simulink library "lib_Gimbal_Ctrl"  (R2019a)
settings: Solver=VariableStepAuto  StartTime=0.0  StopTime=10.0  RelTol=1e-3
undefined symbols (not defined in the file or in its folder): FT_HWI_CC_Data, HIL_Data, Standard_Devices, UDP_Protocol
libraries: simulink x19, sldrtlib x2
(part 2 of 2)

== system lib_Gimbal_Ctrl/Gimbel_Ctrl/Gimbal_Controller/Controller/Voltage_Limitations/If Action limit_pitch ==
  In1 : Inport
  Action Port : ActionPort
  Limit_Voltage_Pitch : Saturate  UpperLimit=Gimbal_Ctrl.PitchCmdMaxVolt  LowerLimit=-Gimbal_Ctrl.PitchCmdMaxVolt
  Out1 : Outport
  wires:
  In1/1 -> Limit_Voltage_Pitch/1
  Limit_Voltage_Pitch/1 -> Out1/1

== system lib_Gimbal_Ctrl/Gimbel_Ctrl/Gimbal_Controller/Controller/Voltage_Limitations/If Action limit_roll ==
  In1 : Inport
  Action Port : ActionPort
  Limit_Voltage_Roll : Saturate  UpperLimit=Gimbal_Ctrl.RollCmdMaxVolt  LowerLimit=-Gimbal_Ctrl.RollCmdMaxVolt
  Out1 : Outport
  wires:
  In1/1 -> Limit_Voltage_Roll/1
  Limit_Voltage_Roll/1 -> Out1/1

== system lib_Gimbal_Ctrl/Gimbel_Ctrl/Gimbal_Controller/Controller/Voltage_Limitations/If Action limit_yaw ==
  In1 : Inport
  Action Port : ActionPort
  Limit_Voltage_Yaw : Saturate  UpperLimit=Gimbal_Ctrl.YawCmdMaxVolt  LowerLimit=-Gimbal_Ctrl.YawCmdMaxVolt
  Out1 : Outport
  wires:
  In1/1 -> Limit_Voltage_Yaw/1
  Limit_Voltage_Yaw/1 -> Out1/1

== system lib_Gimbal_Ctrl/Gimbel_Ctrl/Gimbal_Controller/Controller/Voltage_Limitations/If Action pass_pitch ==
  In1 : Inport
  Action Port : ActionPort
  Out1 : Outport
  wires:
  In1/1 -> Out1/1

== system lib_Gimbal_Ctrl/Gimbel_Ctrl/Gimbal_Controller/Controller/Voltage_Limitations/If Action pass_roll ==
  In1 : Inport
  Action Port : ActionPort
  Out1 : Outport
  wires:
  In1/1 -> Out1/1

== system lib_Gimbal_Ctrl/Gimbel_Ctrl/Gimbal_Controller/Controller/Voltage_Limitations/If Action pass_yaw ==
  In1 : Inport
  Action Port : ActionPort
  Out1 : Outport
  wires:
  In1/1 -> Out1/1

== system lib_Gimbal_Ctrl/Gimbel_Ctrl/Gimbal_Controller/Controller/Controller_Pitch/Limits/Enabled adapt ==
  vel : Inport
  upper_limit : Inport  Port=2
  lower_limit : Inport  Port=3
  Enable : EnablePort
  Abs : Abs
  Add : Sum  Inputs=+-
  Constant : Constant  Value=Gimbal_Ctrl.Pitch_hard_limit_vel
  Constant1 : Constant  Value=Gimbal_Ctrl.Pitch_limit_adaption_coef-1
  Divide : Product  Inputs=*/
  Gain : Gain  Gain=Gimbal_Ctrl.Pitch_limit_adaption_coef
  Product : Product
  Product1 : Product
  upper_limit_adapted : Outport
  lower_limit_adapted : Outport  Port=2
  wires:
  Constant/1 -> Abs/1
  Abs/1 -> Divide/1
  vel/1 -> Divide/2
  Divide/1 -> Gain/1
  Gain/1 -> Add/1
  Constant1/1 -> Add/2
  upper_limit/1 -> Product/2
  Add/1 -> Product/1, Product1/1
  Product/1 -> upper_limit_adapted/1
  lower_limit/1 -> Product1/2
  Product1/1 -> lower_limit_adapted/1

== system lib_Gimbal_Ctrl/Gimbel_Ctrl/Gimbal_Controller/Controller/Controller_Pitch/Limits/Enabled pass ==
  upper_limit : Inport
  lower_limit : Inport  Port=2
  Enable : EnablePort
  upper_limit_pass : Outport
  lower_limit_pass : Outport  Port=2
  wires:
  upper_limit/1 -> upper_limit_pass/1
  lower_limit/1 -> lower_limit_pass/1

== system lib_Gimbal_Ctrl/Gimbel_Ctrl/Gimbal_Controller/Controller/Controller_Pitch/PID_Controller_Dynamic_Limits/Saturation ==
  upper_limit : Inport
  lower_limit : Inport  Port=2
  in : Inport  Port=3
  Enable : EnablePort
  Saturation Dynamic : simulink/Discontinuities/Saturation Dynamic  OutMin=[]  OutMax=[]  OutDataTypeStr=Inherit: Same as second input  OutDataType=fixdt(1, 16)  OutScaling=2^-10  DoSatur=off
  out : Outport
  wires:
  in/1 -> Saturation Dynamic/2
  Saturation Dynamic/1 -> out/1
  lower_limit/1 -> Saturation Dynamic/3
  upper_limit/1 -> Saturation Dynamic/1

== system lib_Gimbal_Ctrl/Gimbel_Ctrl/Gimbal_Controller/Controller/Controller_Pitch/PID_Controller_Dynamic_Limits/pass ==
  in : Inport
  Enable : EnablePort
  out : Outport
  wires:
  in/1 -> out/1

== system lib_Gimbal_Ctrl/Gimbel_Ctrl/Gimbal_Controller/Controller/Controller_Roll/Limits/Enabled adapt ==
  vel : Inport
  upper_limit : Inport  Port=2
  lower_limit : Inport  Port=3
  Enable : EnablePort
  Abs : Abs
  Add : Sum  Inputs=+-
  Constant : Constant  Value=Gimbal_Ctrl.Roll_hard_limit_vel
  Constant1 : Constant  Value=Gimbal_Ctrl.Roll_limit_adaption_coef-1
  Divide : Product  Inputs=*/
  Gain : Gain  Gain=Gimbal_Ctrl.Roll_limit_adaption_coef
  Product : Product
  Product1 : Product
  upper_limit_adapted : Outport
  lower_limit_adapted : Outport  Port=2
  wires:
  Constant/1 -> Abs/1
  Abs/1 -> Divide/1
  vel/1 -> Divide/2
  Divide/1 -> Gain/1
  Gain/1 -> Add/1
  Constant1/1 -> Add/2
  upper_limit/1 -> Product/2
  Add/1 -> Product/1, Product1/1
  Product/1 -> upper_limit_adapted/1
  lower_limit/1 -> Product1/2
  Product1/1 -> lower_limit_adapted/1

== system lib_Gimbal_Ctrl/Gimbel_Ctrl/Gimbal_Controller/Controller/Controller_Roll/Limits/Enabled pass ==
  upper_limit : Inport
  lower_limit : Inport  Port=2
  Enable : EnablePort
  upper_limit_pass : Outport
  lower_limit_pass : Outport  Port=2
  wires:
  upper_limit/1 -> upper_limit_pass/1
  lower_limit/1 -> lower_limit_pass/1

== system lib_Gimbal_Ctrl/Gimbel_Ctrl/Gimbal_Controller/Controller/Controller_Roll/PID_Controller_Dynamic_Limits/Saturation ==
  upper_limit : Inport
  lower_limit : Inport  Port=2
  in : Inport  Port=3
  Enable : EnablePort
  Saturation Dynamic : simulink/Discontinuities/Saturation Dynamic  OutMin=[]  OutMax=[]  OutDataTypeStr=Inherit: Same as second input  OutDataType=fixdt(1, 16)  OutScaling=2^-10  DoSatur=off
  out : Outport
  wires:
  in/1 -> Saturation Dynamic/2
  Saturation Dynamic/1 -> out/1
  lower_limit/1 -> Saturation Dynamic/3
  upper_limit/1 -> Saturation Dynamic/1

== system lib_Gimbal_Ctrl/Gimbel_Ctrl/Gimbal_Controller/Controller/Controller_Roll/PID_Controller_Dynamic_Limits/pass ==
  in : Inport
  Enable : EnablePort
  out : Outport
  wires:
  in/1 -> out/1

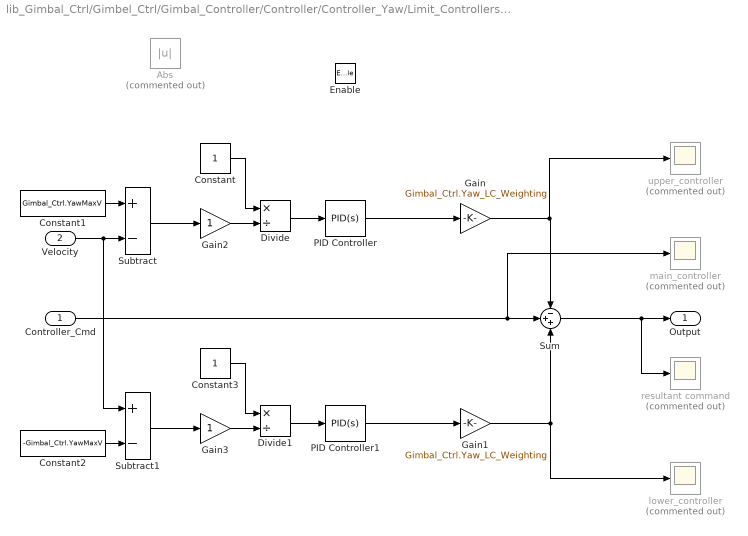
== system lib_Gimbal_Ctrl/Gimbel_Ctrl/Gimbal_Controller/Controller/Controller_Yaw/Limit_Controllers/Control_Limits ==
  Controller_Cmd : Inport
  Velocity : Inport  Port=2
  Enable : EnablePort
  Abs : Abs  Commented=on
  Constant : Constant
  Constant1 : Constant  Value=Gimbal_Ctrl.YawMaxV
  Constant2 : Constant  Value=-Gimbal_Ctrl.YawMaxV
  Constant3 : Constant
  Divide : Product  Inputs=*/
  Divide1 : Product  Inputs=*/
  Gain : Gain  Gain=Gimbal_Ctrl.Yaw_LC_Weighting
  Gain1 : Gain  Gain=Gimbal_Ctrl.Yaw_LC_Weighting
  Gain2 : Gain
  Gain3 : Gain
  PID Controller : simulink/Continuous/PID Controller  Controller=PID  Form=Parallel  TimeDomain=Continuous-time  SampleTime=-1  IntegratorMethod=Forward Euler  FilterMethod=Forward Euler  ControllerParametersSource=internal  P=Gimbal_Ctrl.Yaw_LC_Proportional_Gain  I=Gimbal_Ctrl.Yaw_LC_Integral_Gain  D=Gimbal_Ctrl.Yaw_LC_Derivative_Gain  UseFilter=on  N=100  TunerSelectOption=Transfer Function Based (PID Tuner App)  InitialConditionSource=internal  InitialConditionForIntegrator=0  InitialConditionForFilter=0  DifferentiatorICPrevScaledInput=0  ExternalReset=none  TrackingMode=off  Kt=1  LimitOutput=on  UpperSaturationLimit=20  LowerSaturationLimit=-20  LinearizeAsGain=on  AntiWindupMode=back-calculation  Kb=1  POutMin=[]  POutMax=[]  IOutMin=[]  IOutMax=[]  DOutMin=[]  DOutMax=[]  NOutMin=[]  NOutMax=[]  SumOutMin=[]  SumOutMax=[]  SaturationOutMin=[]  SaturationOutMax=[]  PParamMin=[]  PParamMax=[]  IParamMin=[]  IParamMax=[]  DParamMin=[]  DParamMax=[]  NParamMin=[]  NParamMax=[]  KbParamMin=[]  KbParamMax=[]  KtParamMin=[]  KtParamMax=[]  KbOutMin=[]  KbOutMax=[]  KtOutMin=[]  KtOutMax=[]  IntegratorOutMin=[]  IntegratorOutMax=[]  FilterOutMin=[]  FilterOutMax=[]  SumI1OutMin=[]  SumI1OutMax=[]  SumI2OutMin=[]  SumI2OutMax=[]  SumI3OutMin=[]  SumI3OutMax=[]  SumI4OutMin=[]  SumI4OutMax=[]  SumDOutMin=[]  SumDOutMax=[]  DifferentiatorOutMin=[]  DifferentiatorOutMax=[]  FilterDiffOutCoefMin=[]  FilterDiffOutCoefMax=[]  ReciprocalOutMin=[]  ReciprocalOutMax=[]  SumDenOutMin=[]  SumDenOutMax=[]  SumNumOutMin=[]  SumNumOutMax=[]  DivideOutMin=[]  DivideOutMax=[]  IntegratorContinuousStateAttributes=''  IntegratorStateMustResolveToSignalObject=off  IntegratorRTWStateStorageClass=Auto  FilterContinuousStateAttributes=''  FilterStateMustResolveToSignalObject=off  FilterRTWStateStorageClass=Auto  ParallelPVariant=InternalParameters  IdealPVariant=Disabled  IVariant=InternalParameters  DVariant=InternalParameters  IntegratorVariant=Continuous  SatVariant=Enabled  AWVariant=BackCalculation  PCopyVariant=Disabled  TRVariant=Disabled  FdbkBlocksVariant=Forward  IdealPFdbkVariant=Disabled  SatFdbkVariant=Disabled  DerivativeFilterVariant=ContFilter  NVariant=InternalParameters  NCopyVariant=Disabled  FilterICVariant=InternalICsFilter  IntegratorICVariant=InternalICs  ExternalResetVariant=Disabled  TRSumVariant=Passthrough  SumFdbkVariant=Disabled  SumVariant=Sum_PID
  PID Controller1 : simulink/Continuous/PID Controller  Controller=PID  Form=Parallel  TimeDomain=Continuous-time  SampleTime=-1  IntegratorMethod=Forward Euler  FilterMethod=Forward Euler  ControllerParametersSource=internal  P=Gimbal_Ctrl.Yaw_LC_Proportional_Gain  I=Gimbal_Ctrl.Yaw_LC_Integral_Gain  D=Gimbal_Ctrl.Yaw_LC_Derivative_Gain  UseFilter=on  N=100  TunerSelectOption=Transfer Function Based (PID Tuner App)  InitialConditionSource=internal  InitialConditionForIntegrator=0  InitialConditionForFilter=0  DifferentiatorICPrevScaledInput=0  ExternalReset=none  TrackingMode=off  Kt=1  LimitOutput=on  UpperSaturationLimit=20  LowerSaturationLimit=-20  LinearizeAsGain=off  AntiWindupMode=back-calculation  Kb=1  POutMin=[]  POutMax=[]  IOutMin=[]  IOutMax=[]  DOutMin=[]  DOutMax=[]  NOutMin=[]  NOutMax=[]  SumOutMin=[]  SumOutMax=[]  SaturationOutMin=[]  SaturationOutMax=[]  PParamMin=[]  PParamMax=[]  IParamMin=[]  IParamMax=[]  DParamMin=[]  DParamMax=[]  NParamMin=[]  NParamMax=[]  KbParamMin=[]  KbParamMax=[]  KtParamMin=[]  KtParamMax=[]  KbOutMin=[]  KbOutMax=[]  KtOutMin=[]  KtOutMax=[]  IntegratorOutMin=[]  IntegratorOutMax=[]  FilterOutMin=[]  FilterOutMax=[]  SumI1OutMin=[]  SumI1OutMax=[]  SumI2OutMin=[]  SumI2OutMax=[]  SumI3OutMin=[]  SumI3OutMax=[]  SumI4OutMin=[]  SumI4OutMax=[]  SumDOutMin=[]  SumDOutMax=[]  DifferentiatorOutMin=[]  DifferentiatorOutMax=[]  FilterDiffOutCoefMin=[]  FilterDiffOutCoefMax=[]  ReciprocalOutMin=[]  ReciprocalOutMax=[]  SumDenOutMin=[]  SumDenOutMax=[]  SumNumOutMin=[]  SumNumOutMax=[]  DivideOutMin=[]  DivideOutMax=[]  IntegratorContinuousStateAttributes=''  IntegratorStateMustResolveToSignalObject=off  IntegratorRTWStateStorageClass=Auto  FilterContinuousStateAttributes=''  FilterStateMustResolveToSignalObject=off  FilterRTWStateStorageClass=Auto  ParallelPVariant=InternalParameters  IdealPVariant=Disabled  IVariant=InternalParameters  DVariant=InternalParameters  IntegratorVariant=Continuous  SatVariant=Enabled  AWVariant=BackCalculation  PCopyVariant=Disabled  TRVariant=Disabled  FdbkBlocksVariant=Forward  IdealPFdbkVariant=Disabled  SatFdbkVariant=Disabled  DerivativeFilterVariant=ContFilter  NVariant=InternalParameters  NCopyVariant=Disabled  FilterICVariant=InternalICsFilter  IntegratorICVariant=InternalICs  ExternalResetVariant=Disabled  TRSumVariant=Passthrough  SumFdbkVariant=Disabled  SumVariant=Sum_PID
  Subtract : Sum  Inputs=+-
  Subtract1 : Sum  Inputs=+-
  Sum : Sum  Inputs=-++
  lower_controller : Scope  Commented=on
  main_controller : Scope  Commented=on
  resultant command : Scope  Commented=on
  upper_controller : Scope  Commented=on
  Output : Outport
  wires:
  Sum/1 -> resultant command/1, Output/1
  Gain/1 -> upper_controller/1, Sum/1
  Gain1/1 -> lower_controller/1, Sum/3
  Controller_Cmd/1 -> main_controller/1, Sum/2
  Constant1/1 -> Subtract/1
  Velocity/1 -> Subtract1/1, Subtract/2
  Subtract/1 -> Gain2/1
  Constant/1 -> Divide/1
  Divide/1 -> PID Controller/1
  Constant2/1 -> Subtract1/2
  Subtract1/1 -> Gain3/1
  Constant3/1 -> Divide1/1
  Divide1/1 -> PID Controller1/1
  PID Controller/1 -> Gain/1
  PID Controller1/1 -> Gain1/1
  Gain3/1 -> Divide1/2
  Gain2/1 -> Divide/2

== system lib_Gimbal_Ctrl/Gimbel_Ctrl/Gimbal_Controller/Controller/Controller_Yaw/Limit_Controllers/pass ==
  Controller_Cmd : Inport
  Enable : EnablePort
  Output : Outport
  wires:
  Controller_Cmd/1 -> Output/1

== system lib_Gimbal_Ctrl/Gimbel_Ctrl/Gimbal_Controller/Controller/Controller_Yaw/Limits/Enabled adapt ==
  vel : Inport
  upper_limit : Inport  Port=2
  lower_limit : Inport  Port=3
  Enable : EnablePort
  Abs : Abs
  Add : Sum  Inputs=+-
  Constant : Constant  Value=Gimbal_Ctrl.Yaw_hard_limit_vel
  Constant1 : Constant  Value=Gimbal_Ctrl.Yaw_limit_adaption_coef-1
  Divide : Product  Inputs=*/
  Gain : Gain  Gain=Gimbal_Ctrl.Yaw_limit_adaption_coef
  Product : Product
  Product1 : Product
  upper_limit_adapted : Outport
  lower_limit_adapted : Outport  Port=2
  wires:
  Constant/1 -> Abs/1
  Abs/1 -> Divide/1
  vel/1 -> Divide/2
  Divide/1 -> Gain/1
  Gain/1 -> Add/1
  Constant1/1 -> Add/2
  upper_limit/1 -> Product/2
  Add/1 -> Product/1, Product1/1
  Product/1 -> upper_limit_adapted/1
  lower_limit/1 -> Product1/2
  Product1/1 -> lower_limit_adapted/1

== system lib_Gimbal_Ctrl/Gimbel_Ctrl/Gimbal_Controller/Controller/Controller_Yaw/Limits/Enabled pass ==
  upper_limit : Inport
  lower_limit : Inport  Port=2
  Enable : EnablePort
  upper_limit_pass : Outport
  lower_limit_pass : Outport  Port=2
  wires:
  upper_limit/1 -> upper_limit_pass/1
  lower_limit/1 -> lower_limit_pass/1

== system lib_Gimbal_Ctrl/Gimbel_Ctrl/Gimbal_Controller/Controller/Controller_Yaw/PID_Controller_Dynamic_Limits/Saturation ==
  upper_limit : Inport
  lower_limit : Inport  Port=2
  in : Inport  Port=3
  Enable : EnablePort
  Saturation Dynamic : simulink/Discontinuities/Saturation Dynamic  OutMin=[]  OutMax=[]  OutDataTypeStr=Inherit: Same as second input  OutDataType=fixdt(1, 16)  OutScaling=2^-10  DoSatur=off
  out : Outport
  wires:
  in/1 -> Saturation Dynamic/2
  Saturation Dynamic/1 -> out/1
  lower_limit/1 -> Saturation Dynamic/3
  upper_limit/1 -> Saturation Dynamic/1

== system lib_Gimbal_Ctrl/Gimbel_Ctrl/Gimbal_Controller/Controller/Controller_Yaw/PID_Controller_Dynamic_Limits/pass ==
  in : Inport
  Enable : EnablePort
  out : Outport
  wires:
  in/1 -> out/1

== system lib_Gimbal_Ctrl/Gimbel_Ctrl/Gimbal_Controller/Controller/Monitor_Velocity_Limits/Pitch_rate_limit/If Action Subsystem ==
  In1 : Inport
  Action Port : ActionPort
  Out1 : Outport
  wires:
  In1/1 -> Out1/1

== system lib_Gimbal_Ctrl/Gimbel_Ctrl/Gimbal_Controller/Controller/Monitor_Velocity_Limits/Pitch_rate_limit/If Action Subsystem1 ==
  In1 : Inport
  Action Port : ActionPort
  Out1 : Outport
  wires:
  In1/1 -> Out1/1

== system lib_Gimbal_Ctrl/Gimbel_Ctrl/Gimbal_Controller/Controller/Monitor_Velocity_Limits/Roll_Rate_limit/If Action Subsystem ==
  In1 : Inport
  Action Port : ActionPort
  Out1 : Outport
  wires:
  In1/1 -> Out1/1

== system lib_Gimbal_Ctrl/Gimbel_Ctrl/Gimbal_Controller/Controller/Monitor_Velocity_Limits/Roll_Rate_limit/If Action Subsystem1 ==
  In1 : Inport
  Action Port : ActionPort
  Out1 : Outport
  wires:
  In1/1 -> Out1/1

== system lib_Gimbal_Ctrl/Gimbel_Ctrl/Gimbal_Controller/Controller/Monitor_Velocity_Limits/Yaw_rate_limit/If Action Subsystem ==
  In1 : Inport
  Action Port : ActionPort
  Out1 : Outport
  wires:
  In1/1 -> Out1/1

== system lib_Gimbal_Ctrl/Gimbel_Ctrl/Gimbal_Controller/Controller/Monitor_Velocity_Limits/Yaw_rate_limit/If Action Subsystem1 ==
  In1 : Inport
  Action Port : ActionPort
  Out1 : Outport
  wires:
  In1/1 -> Out1/1
